simulink model "MSD"  (R2024a)
settings: Solver=VariableStepAuto  StartTime=0.0  StopTime=10.0  RelTol=1e-3
model workspace (MATLAB code in the model file):
  | m=1;
  | k=2;
  | c=2;
settings Model: Creator=User  LastModifiedBy=User

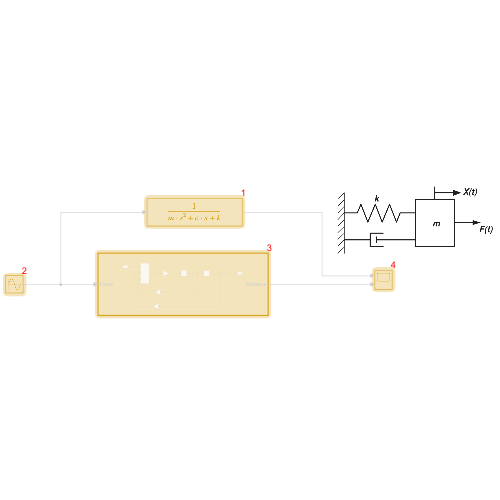
[thumbnail: Simulink's stored preview of the top-level diagram]
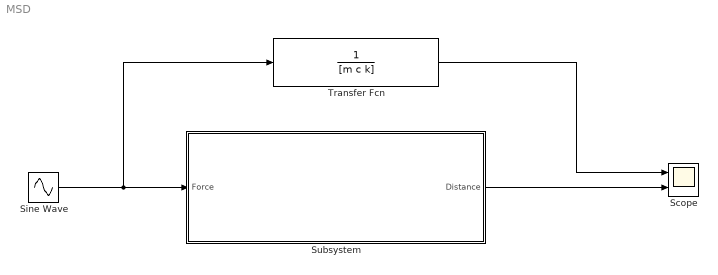
== system MSD ==
  Scope : Scope  NumInputPorts=2
  Sine Wave : Sin  SampleTime=0
  Subsystem : Subsystem  TreatAsAtomicUnit=on
  Transfer Fcn : TransferFcn  Denominator=[m c k]
  wires:
  Sine Wave/1 -> Transfer Fcn/1, Subsystem/1(Force)
  Transfer Fcn/1 -> Scope/1
  Subsystem/1(Distance) -> Scope/2

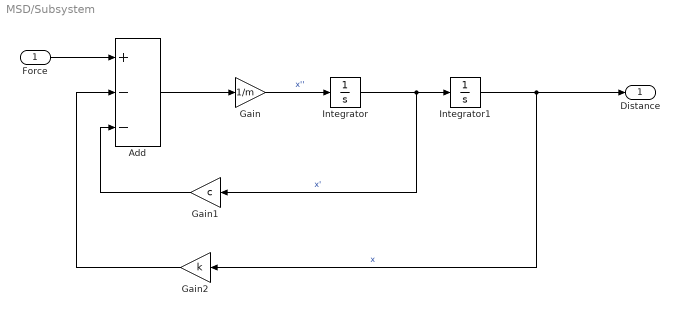
== system MSD/Subsystem ==
  Force : Inport
  Add : Sum  Inputs=+--
  Gain : Gain  Gain=1/m
  Gain1 : Gain  Gain=c
  Gain2 : Gain  Gain=k
  Integrator : Integrator
  Integrator1 : Integrator
  Distance : Outport
  wires:
  Add/1 -> Gain/1
  Integrator/1 -> Gain1/1, Integrator1/1  "x'"
  Gain1/1 -> Add/3
  Gain/1 -> Integrator/1  "x''"
  Force/1 -> Add/1
  Gain2/1 -> Add/2
  Integrator1/1 -> Gain2/1, Distance/1  "x"
